simulink model "IEEE13bus_1subsystem"  (R2022b)
settings: Solver=ode4  StartTime=0.0  StopTime=inf  FixedStep=Ts  MaxStep=1e-4  RelTol=1e-4
InitFcn:
  | a=1; % Loading Factor
  | Ts=50e-6;
  | % phase to sequence conversion of RXB matrices
  | c=1*exp(sqrt(-1)*(120*pi/180));
  | T=[1 1 1;1 c*c c;1 c c*c];
  | Tinv=1/3*[1 1 1;1 c c*c;1 c*c c];
  | 
  | % Simulation data for the IEEE 13 Node Test Feeder model
  | mi2km = 1.60934;%  miles to km conversion
  | ft2km = 0.0003048; % feet to km conversion
  | ms2F = 1*1e-6/(2*pi*60);% microsiemens to Farads conversion
  | 
  | 
  | %% Configuration 601
  | % Series Resitance and Reactance - ohm/mile
  | R_601 = [0.3465 0.1560 0.1580;0.1560 0.3375 0.1535;0.1580 0.1535 0.3414];
  | X_601 = [1.1079 0.5017 0.4236;0.5017 1.0478 0.3849;0.4236 0.3849 1.0348];
  | % charging susceptance - microsiemens/mile
  | B_601 = [6.2998 -1.9958 -1.2595;-1.9958 5.9597 -0.7417;-1.2595 -0.7417 5.6386];
  | 
  | R_601 = R_601/mi2km;
  | Rseq=Tinv*R_601*T;
  | R1_601=Rseq(2,2);R0_601=Rseq(1,1);
  | 
  | L_601 = (X_601/(2*pi*60))/mi2km;
  | Lseq=Tinv*L_601*T;
  | L1_601=Lseq(2,2);L0_601=Lseq(1,1);
  | 
  | C_601 =(B_601*ms2F)/mi2km;
  | Cseq=Tinv*C_601*T;
  | C1_601=Cseq(2,2);C0_601=Cseq(1,1);
  | 
  | %% Configuration 602 - series reactance - ohm/mile
  | R_602 = [0.7526 0.1580 0.1560;0.1580 0.7475 0.1535;0.1560 0.1535 0.7436];
  | X_602 = [1.1814 0.4236 0.5017;0.4236 1.1983 0.3849;0.5017 0.3849 1.2112];
  | % charging susceptance - microsiemens/mile
  | B_602 = [5.6990 -1.0817 -1.6905;-1.0817 5.1795 -0.6588;-1.6905 -0.6588 5.4246];
  | 
  | R_602 = R_602/mi2km;
  | Rseq=Tinv*R_602*T;
  | R1_602=Rseq(2,2);R0_602=Rseq(1,1);
  | 
  | L_602 = (X_602/(2*pi*60))/mi2km;
  | Lseq=Tinv*L_602*T;
  | L1_602=Lseq(2,2);L0_602=Lseq(1,1);
  | 
  | C_602 =(B_602*ms2F)/mi2km;
  | Cseq=Tinv*C_602*T;
  | C1_602=Cseq(2,2);C0_602=Cseq(1,1);
  | %% Configuration 603 - series reactance - ohm/mile
  | R_603 = [0 0 0;0 1.3294 0.2066;0 0.2066 1.3238];
  | X_603 = [0 0 0;0 1.3471 0.4591;0 0.4591 1.3569];
  | % charging susceptance - microsiemens/mile
  | B_603 = [0 0 0;0 4.7097 -0.8999;0 -0.8999 4.6658];
  | 
  | % convert for SPS
  | R_603 = R_603/mi2km;
  | Rseq=Tinv*R_603*T;
  | R1_603=Rseq(2,2);R0_603=Rseq(1,1);
  | 
  | ... (+71 lines)
undefined symbols (not defined in the file): find_system, I, Left, MOV_segment9, powergui, Right, type, V, X
libraries: spsSeriesRLCBranchLib x57, spsGroundLib x42, spsVoltageMeasurementLib x18, spsThreePhaseVIMeasurementLib x16, spsDCVoltageSourceLib x12, spsThreePhaseSeriesRLCLoadLib x7, ssn_lib x6, spsACCurrentSourceLib x6, spsOnDelayLib x6, spsThreePhasePISectionLineLib x5, spsSeriesRLCLoadLib x5, spsRMSLib x4
(part 2 of 4)

== system IEEE13bus_1subsystem/SM_13p/Regulator 1 ==
  Mux : Mux  Inputs=3
  Single Phase SVR_A : Subsystem  LoadFcn=find_system(gcs,'FollowLinks', 'on', 'LookUnderMasks', 'all');  mask(Single-Phase OLTC){pNom=5e6/3, fNom=60, vNom=4160/sqrt(3), ctRatio=700, ptRatio=20, DeltaU=0.00625, TapMinMax=[-16 16], InitialTap=10, TapSelectionTime=0.2, RegulatorOn=on, Regulator=[122/120  2/120  0.2], Comp=[3 9]}
      mask prompts: pNom "Nominal Power (VA)"; fNom "Nominal Frequency (Hz)"; vNom "Nominal Voltage (Vrms)"; ctRatio "Primary CT Rating (A)"; ptRatio "PT Ratio"; DeltaU "Voltage Step Per Tap (pu)"; TapMinMax "Minimum and Maximum Tap Positions"; InitialTap "Initial Tap Position"; TapSelectionTime "Tap Selection Time (s)"; RegulatorOn "Voltage Regulator"; Regulator "Voltage Regulator [ Vref(pu) DeadBand(pu)  Delay(s)]"; Comp "Compensator Settings [R (V) X(V)]"
      mask help:
      | Models a single-phase On Load Tap Changer (OLTC). The single-phase secondary of multi-tap winding is modeled with a Variable-Ratio Transformer block.
      |
      | The transformer voltage ratio U2/U1 (in pu) is given by:
      |                 U2/U1= 1+TapPosition*DeltaU
      | Tap position 0 corresponds to nominal voltage ratio.
      |
      | When Voltage regulator is 'on',  voltage regulator asks for a tap change if:
      |                  abs(Vm-Vref)>DeadBand/2  during a time  t > Delay.
      |
      | where 'Vm' is voltage measured at regulating point and Vref is reference voltage.
      | With line drop compensation, Vm=Vsec-Isec(R+jX)
      mask init:
      | RegulatorVref=Regulator(1);
      | RegulatorDeadBand=Regulator(2);
      | RegulatorDelay=Regulator(3);
      | Rc=Comp(1);
      | Xc=Comp(2);
      mask TypeOptions RegulatorOn: off | on
      mask Callback RegulatorOn:
      | tempMaskVis=get_param(gcb,'MaskVisibilities');
      | if strcmp(get_param(gcb,'RegulatorOn'),'on')
      | 	tempMaskVis{11}='on';
      | 	set_param(gcb,'MaskVisibilities',tempMaskVis);
      | else
      | 	tempMaskVis{11}='off';
      | 	set_param(gcb,'MaskVisibilities',tempMaskVis);
      | end
      | if strcmp(get_param(gcb,'RegulatorOn'),'on')
      | 	tempMaskVis{12}='on';
      | 	set_param(gcb,'MaskVisibilities',tempMaskVis);
      | else
      | 	tempMaskVis{12}='off';
      | 	set_param(gcb,'MaskVisibilities',tempMaskVis);
      | end
      mask DialogControl Container8 Prompt: Setup
      mask DialogControl Container13 Prompt: Regulator Parameters
      mask Display:
      | color('green');
      | r=50;x=40;y=80;
      | th = 0:pi/100:2*pi;
      | f = r * exp(j*th) + x+j*y;
      | plot(real(f), imag(f));
      | color('blue');
      | plot([-10 90],[30,130])
      | plot([75 90],[125,130])
      | plot([85 90],[115,130])
      | color('black')
      | port_label('Lconn',1,'S');port_label('Rconn',1,'L');
      | text(58,115,'Tap');
      | text(43,70,'Vsec');
      | text(48,95,'Isec');
  Single Phase SVR_A1 : Subsystem  LoadFcn=find_system(gcs,'FollowLinks', 'on', 'LookUnderMasks', 'all');  mask(Single-Phase OLTC){pNom=5e6/3, fNom=60, vNom=4160/sqrt(3), ctRatio=700, ptRatio=20, DeltaU=0.00625, TapMinMax=[-16 16], InitialTap=8, TapSelectionTime=0.2, RegulatorOn=on, Regulator=[122/120  2/120  0.2], Comp=[3 9]}
      mask prompts: pNom "Nominal Power (VA)"; fNom "Nominal Frequency (Hz)"; vNom "Nominal Voltage (Vrms)"; ctRatio "Primary CT Rating (A)"; ptRatio "PT Ratio"; DeltaU "Voltage Step Per Tap (pu)"; TapMinMax "Minimum and Maximum Tap Positions"; InitialTap "Initial Tap Position"; TapSelectionTime "Tap Selection Time (s)"; RegulatorOn "Voltage Regulator"; Regulator "Voltage Regulator [ Vref(pu) DeadBand(pu)  Delay(s)]"; Comp "Compensator Settings [R (V) X(V)]"
      mask help:
      | Models a single-phase On Load Tap Changer (OLTC). The single-phase secondary of multi-tap winding is modeled with a Variable-Ratio Transformer block.
      |
      | The transformer voltage ratio U2/U1 (in pu) is given by:
      |                 U2/U1= 1+TapPosition*DeltaU
      | Tap position 0 corresponds to nominal voltage ratio.
      |
      | When Voltage regulator is 'on',  voltage regulator asks for a tap change if:
      |                  abs(Vm-Vref)>DeadBand/2  during a time  t > Delay.
      |
      | where 'Vm' is voltage measured at regulating point and Vref is reference voltage.
      | With line drop compensation, Vm=Vsec-Isec(R+jX)
      mask init:
      | RegulatorVref=Regulator(1);
      | RegulatorDeadBand=Regulator(2);
      | RegulatorDelay=Regulator(3);
      | Rc=Comp(1);
      | Xc=Comp(2);
      mask TypeOptions RegulatorOn: off | on
      mask Callback RegulatorOn:
      | tempMaskVis=get_param(gcb,'MaskVisibilities');
      | if strcmp(get_param(gcb,'RegulatorOn'),'on')
      | 	tempMaskVis{11}='on';
      | 	set_param(gcb,'MaskVisibilities',tempMaskVis);
      | else
      | 	tempMaskVis{11}='off';
      | 	set_param(gcb,'MaskVisibilities',tempMaskVis);
      | end
      | if strcmp(get_param(gcb,'RegulatorOn'),'on')
      | 	tempMaskVis{12}='on';
      | 	set_param(gcb,'MaskVisibilities',tempMaskVis);
      | else
      | 	tempMaskVis{12}='off';
      | 	set_param(gcb,'MaskVisibilities',tempMaskVis);
      | end
      mask DialogControl Container8 Prompt: Setup
      mask DialogControl Container13 Prompt: Regulator Parameters
      mask Display:
      | color('green');
      | r=50;x=40;y=80;
      | th = 0:pi/100:2*pi;
      | f = r * exp(j*th) + x+j*y;
      | plot(real(f), imag(f));
      | color('blue');
      | plot([-10 90],[30,130])
      | plot([75 90],[125,130])
      | plot([85 90],[115,130])
      | color('black')
      | port_label('Lconn',1,'S');port_label('Rconn',1,'L');
      | text(58,115,'Tap');
      | text(43,70,'Vsec');
      | text(48,95,'Isec');
  Single Phase SVR_A2 : Subsystem  LoadFcn=find_system(gcs,'FollowLinks', 'on', 'LookUnderMasks', 'all');  mask(Single-Phase OLTC){pNom=5e6/3, fNom=60, vNom=4160/sqrt(3), ctRatio=700, ptRatio=20, DeltaU=0.00625, TapMinMax=[-16 16], InitialTap=11, TapSelectionTime=0.2, RegulatorOn=on, Regulator=[122/120  2/120  0.2], Comp=[3 9]}
      mask prompts: pNom "Nominal Power (VA)"; fNom "Nominal Frequency (Hz)"; vNom "Nominal Voltage (Vrms)"; ctRatio "Primary CT Rating (A)"; ptRatio "PT Ratio"; DeltaU "Voltage Step Per Tap (pu)"; TapMinMax "Minimum and Maximum Tap Positions"; InitialTap "Initial Tap Position"; TapSelectionTime "Tap Selection Time (s)"; RegulatorOn "Voltage Regulator"; Regulator "Voltage Regulator [ Vref(pu) DeadBand(pu)  Delay(s)]"; Comp "Compensator Settings [R (V) X(V)]"
      mask help:
      | Models a single-phase On Load Tap Changer (OLTC). The single-phase secondary of multi-tap winding is modeled with a Variable-Ratio Transformer block.
      |
      | The transformer voltage ratio U2/U1 (in pu) is given by:
      |                 U2/U1= 1+TapPosition*DeltaU
      | Tap position 0 corresponds to nominal voltage ratio.
      |
      | When Voltage regulator is 'on',  voltage regulator asks for a tap change if:
      |                  abs(Vm-Vref)>DeadBand/2  during a time  t > Delay.
      |
      | where 'Vm' is voltage measured at regulating point and Vref is reference voltage.
      | With line drop compensation, Vm=Vsec-Isec(R+jX)
      mask init:
      | RegulatorVref=Regulator(1);
      | RegulatorDeadBand=Regulator(2);
      | RegulatorDelay=Regulator(3);
      | Rc=Comp(1);
      | Xc=Comp(2);
      mask TypeOptions RegulatorOn: off | on
      mask Callback RegulatorOn:
      | tempMaskVis=get_param(gcb,'MaskVisibilities');
      | if strcmp(get_param(gcb,'RegulatorOn'),'on')
      | 	tempMaskVis{11}='on';
      | 	set_param(gcb,'MaskVisibilities',tempMaskVis);
      | else
      | 	tempMaskVis{11}='off';
      | 	set_param(gcb,'MaskVisibilities',tempMaskVis);
      | end
      | if strcmp(get_param(gcb,'RegulatorOn'),'on')
      | 	tempMaskVis{12}='on';
      | 	set_param(gcb,'MaskVisibilities',tempMaskVis);
      | else
      | 	tempMaskVis{12}='off';
      | 	set_param(gcb,'MaskVisibilities',tempMaskVis);
      | end
      mask DialogControl Container8 Prompt: Setup
      mask DialogControl Container13 Prompt: Regulator Parameters
      mask Display:
      | color('green');
      | r=50;x=40;y=80;
      | th = 0:pi/100:2*pi;
      | f = r * exp(j*th) + x+j*y;
      | plot(real(f), imag(f));
      | color('blue');
      | plot([-10 90],[30,130])
      | plot([75 90],[125,130])
      | plot([85 90],[115,130])
      | color('black')
      | port_label('Lconn',1,'S');port_label('Rconn',1,'L');
      | text(58,115,'Tap');
      | text(43,70,'Vsec');
      | text(48,95,'Isec');
  A : PMIOPort  Side=Left
  a : PMIOPort  Port=2  Side=Right
  B : PMIOPort  Port=3  Side=Left
  b : PMIOPort  Port=4  Side=Right
  C : PMIOPort  Port=5  Side=Left
  c : PMIOPort  Port=6  Side=Right
  Tap : Outport
  wires:
  Single Phase SVR_A/1(Tap) -> Mux/1
  Single Phase SVR_A1/1(Tap) -> Mux/2
  Single Phase SVR_A2/1(Tap) -> Mux/3
  Mux/1 -> Tap/1
  connections:
  Single Phase SVR_A/RConn1 -- a/RConn1
  Single Phase SVR_A/LConn1 -- A/RConn1
  Single Phase SVR_A1/LConn1 -- B/RConn1
  Single Phase SVR_A1/RConn1 -- b/RConn1
  Single Phase SVR_A2/LConn1 -- C/RConn1
  Single Phase SVR_A2/RConn1 -- c/RConn1

== system IEEE13bus_1subsystem/SM_13p/Regulator Taps  ==
  Band Width : Constant  Value=2
  Band Width1 : Constant  Value=2
  Gain : Gain  Gain=1/2
  Gain2 : Gain  Gain=1/2
  Scope3 : Scope  NumInputPorts=5
  Sum : Sum  Inputs=|++
  Sum1 : Sum  Inputs=|+-
  Tap : Scope
  Vref : Constant  Value=122
  Vref1 : Constant  Value=122
  wires:
  [Rg1] -> Tap/1
  Vref/1 -> Sum/1
  Band Width/1 -> Gain/1
  Gain/1 -> Sum/2
  Gain2/1 -> Sum1/2
  Band Width1/1 -> Gain2/1
  Vref1/1 -> Sum1/1
  Sum/1 -> Scope3/1  "Upper Limit"
  [Vr1a] -> Scope3/2  "Vra"
  [Vr1b] -> Scope3/3  "Vrb"
  [Vr1c] -> Scope3/4  "Vrc"
  Sum1/1 -> Scope3/5  "Lower Limit"

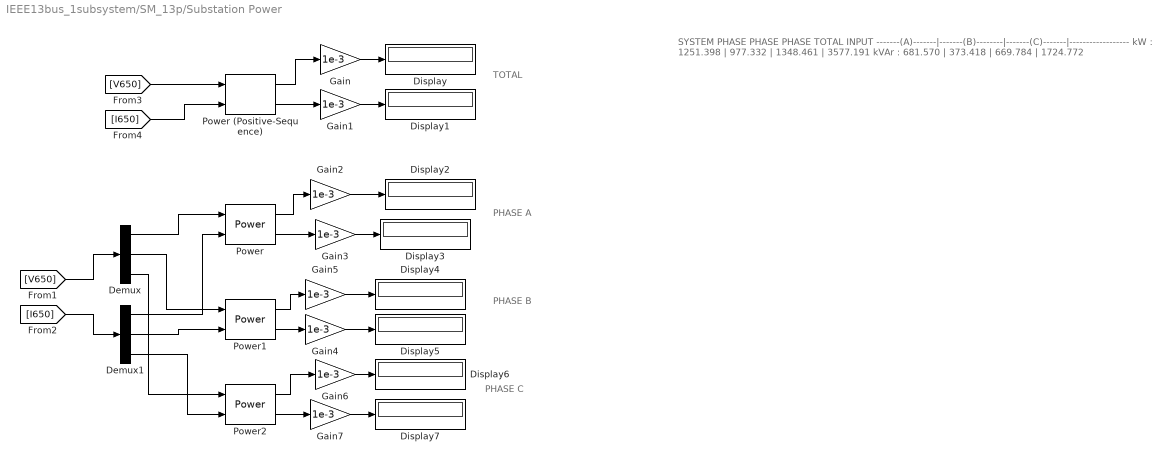
== system IEEE13bus_1subsystem/SM_13p/Substation Power ==
  note: SYSTEM PHASE PHASE PHASE TOTAL
      | INPUT -------(A)-------|-------(B)--------|-------(C)-------|------------------
      | kW : 1251.398 | 977.332 | 1348.461 | 3577.191
      | kVAr : 681.570 | 373.418 | 669.784 | 1724.772
  note: PHASE A
  note: PHASE C
  note: PHASE B
  note: TOTAL
  Demux : Demux  Outputs=3
  Demux1 : Demux  Outputs=3
  Display{,1..7} (8 alike) : Display
  Gain{,1..7} (8 alike) : Gain  Gain=1e-3
  Power : spsPowerLib/Power  Freq=60  Vinit=[1, 0]  Iinit=[1, 0]  Ts=0
  Power (Positive-Sequence) : spsPowerPositiveSequenceLib/Power (Positive-Sequence)  Freq=60  Vinit=[0, 0]  Iinit=[0, 0]  Ts=Ts
      settings: LibrarySourceBlock=|
      | sps_lib/Sensors and Measurements/Power
      | (Positive-Sequence)
  Power1 : spsPowerLib/Power  Freq=60  Vinit=[1, 0]  Iinit=[1, 0]  Ts=0
  Power2 : spsPowerLib/Power  Freq=60  Vinit=[1, 0]  Iinit=[1, 0]  Ts=0
  wires:
  [I650] -> Power (Positive-Sequence)/2
  [V650] -> Power (Positive-Sequence)/1
  Power (Positive-Sequence)/1 -> Gain/1
  Power (Positive-Sequence)/2 -> Gain1/1
  [V650] -> Demux/1
  [I650] -> Demux1/1
  Demux/1 -> Power/1
  Demux1/1 -> Power/2
  Demux/2 -> Power1/1
  Demux1/2 -> Power1/2
  Demux/3 -> Power2/1
  Demux1/3 -> Power2/2
  Power/1 -> Gain2/1
  Power/2 -> Gain3/1
  Power1/1 -> Gain5/1
  Power1/2 -> Gain4/1
  Power2/1 -> Gain6/1
  Power2/2 -> Gain7/1
  Gain/1 -> Display/1
  Gain1/1 -> Display1/1
  Gain2/1 -> Display2/1
  Gain3/1 -> Display3/1
  Gain4/1 -> Display5/1
  Gain5/1 -> Display4/1
  Gain6/1 -> Display6/1
  Gain7/1 -> Display7/1

== system IEEE13bus_1subsystem/powergui/EquivalentModel1 ==
  Sources : Subsystem
  State-Space : S-Function  FunctionName=ssn_sfun_v1  Parameters=1,0  SFunctionDeploymentMode=off  EnableBusSupport=off  SFcnStateName=MOV_segment9,MOV_segment9,MOV_segment9,MOV_segment9,MOV_segment9,MOV_segment9,MOV_segment9,MOV_segment9,MOV_segment9,MOV_segment9
      settings: SFcnIsStateOwnerBlock=on
  Yout : Subsystem
  wires:
  State-Space/1 -> Yout/1(v,i)
  Sources/1(u) -> State-Space/1

== system IEEE13bus_1subsystem/powergui/EquivalentModel2 ==
  Sources : Subsystem
  State-Space : S-Function  FunctionName=ssn_sfun_v1  Parameters=2,0  SFunctionDeploymentMode=off  EnableBusSupport=off  SFcnStateName=MOV_segment9,MOV_segment9,MOV_segment9,MOV_segment9,MOV_segment9,MOV_segment9,MOV_segment9,MOV_segment9,MOV_segment9,MOV_segment9
      settings: SFcnIsStateOwnerBlock=on
  Yout : Subsystem
  wires:
  State-Space/1 -> Yout/1(v,i)
  Sources/1(u) -> State-Space/1

== system IEEE13bus_1subsystem/powergui/EquivalentModel3 ==
  Sources : Subsystem
  State-Space : S-Function  FunctionName=ssn_sfun_v1  Parameters=3,0  SFunctionDeploymentMode=off  EnableBusSupport=off  SFcnStateName=MOV_segment9,MOV_segment9,MOV_segment9,MOV_segment9,MOV_segment9,MOV_segment9,MOV_segment9,MOV_segment9,MOV_segment9,MOV_segment9
      settings: SFcnIsStateOwnerBlock=on
  Yout : Subsystem
  wires:
  State-Space/1 -> Yout/1(v,i)
  Sources/1(u) -> State-Space/1

== system IEEE13bus_1subsystem/powergui/EquivalentModel4 ==
  Gates : Subsystem
  Sources : Subsystem
  State-Space : Subsystem
  Status : Subsystem
  Yout : Subsystem
  wires:
  Gates/1(gates) -> State-Space/2(In2)
  Sources/1(u) -> State-Space/1(In1)
  State-Space/2(Out2) -> Status/1(status)
  State-Space/1(Out1) -> Yout/1(v,i)

== system IEEE13bus_1subsystem/SM_13p/Regulator 1/Single Phase SVR_A ==
  Line Drop Compensator : Subsystem
  Transformer with Taps : Subsystem
  Voltage Regulator Control : Subsystem
  S : PMIOPort  Tag=PMCPort  Side=Left
  L : PMIOPort  Tag=PMCPort  Port=2  Side=Right
  Tap : Outport  VectorParamsAs1DForOutWhenUnconnected=off
  tag scope: Vr1a=global
  wires:
  Transformer with Taps/2(Vsec) -> Line Drop Compensator/2(Vsec)
  Transformer with Taps/1(Isec) -> Line Drop Compensator/1(Isec)
  Voltage Regulator Control/1(N) -> Transformer with Taps/1(N)
  Voltage Regulator Control/2(Tap) -> Tap/1
  Line Drop Compensator/1(Vm) -> [Vr1a], Voltage Regulator Control/1(Vm)
  connections:
  Transformer with Taps/LConn1 -- S/RConn1
  Transformer with Taps/RConn1 -- L/RConn1

== system IEEE13bus_1subsystem/SM_13p/Regulator 1/Single Phase SVR_A1 ==
  Line Drop Compensator : Subsystem
  Transformer with Taps : Subsystem
  Voltage Regulator Control : Subsystem
  S : PMIOPort  Tag=PMCPort  Side=Left
  L : PMIOPort  Tag=PMCPort  Port=2  Side=Right
  Tap : Outport  VectorParamsAs1DForOutWhenUnconnected=off
  tag scope: Vr1b=global
  wires:
  Line Drop Compensator/1(Vm) -> Voltage Regulator Control/1(Vm), [Vr1b]
  Voltage Regulator Control/2(Tap) -> Tap/1
  Voltage Regulator Control/1(N) -> Transformer with Taps/1(N)
  Transformer with Taps/1(Isec) -> Line Drop Compensator/1(Isec)
  Transformer with Taps/2(Vsec) -> Line Drop Compensator/2(Vsec)
  connections:
  Transformer with Taps/RConn1 -- L/RConn1
  Transformer with Taps/LConn1 -- S/RConn1

== system IEEE13bus_1subsystem/SM_13p/Regulator 1/Single Phase SVR_A2 ==
  Line Drop Compensator : Subsystem
  Transformer with Taps : Subsystem
  Voltage Regulator Control : Subsystem
  S : PMIOPort  Tag=PMCPort  Side=Left
  L : PMIOPort  Tag=PMCPort  Port=2  Side=Right
  Tap : Outport  VectorParamsAs1DForOutWhenUnconnected=off
  tag scope: Vr1c=global
  wires:
  Transformer with Taps/2(Vsec) -> Line Drop Compensator/2(Vsec)
  Transformer with Taps/1(Isec) -> Line Drop Compensator/1(Isec)
  Voltage Regulator Control/1(N) -> Transformer with Taps/1(N)
  Voltage Regulator Control/2(Tap) -> Tap/1
  Line Drop Compensator/1(Vm) -> [Vr1c], Voltage Regulator Control/1(Vm)
  connections:
  Transformer with Taps/LConn1 -- S/RConn1
  Transformer with Taps/RConn1 -- L/RConn1

== system IEEE13bus_1subsystem/powergui/EquivalentModel1/Sources ==
  Mux : Mux  Inputs=[1 1]
  u : Outport  VectorParamsAs1DForOutWhenUnconnected=off
  wires:
  Mux/1 -> u/1
  [T91_7966_12561094007631] -> Mux/1
  [T91_7953_12480495761568] -> Mux/2

== system IEEE13bus_1subsystem/powergui/EquivalentModel1/Yout ==
  v,i : Inport
  Demux : Demux  Outputs=1
  tag scope: T94_8498_15482413429189=global
  wires:
  v,i/1 -> Demux/1
  Demux/1 -> [T94_8498_15482413429189]

== system IEEE13bus_1subsystem/powergui/EquivalentModel2/Sources ==
  Mux : Mux  Inputs=[1 1]
  u : Outport  VectorParamsAs1DForOutWhenUnconnected=off
  wires:
  Mux/1 -> u/1
  [T92_8015_12801519000204] -> Mux/1
  [T92_8002_12718661753869] -> Mux/2

== system IEEE13bus_1subsystem/powergui/EquivalentModel2/Yout ==
  v,i : Inport
  Demux : Demux  Outputs=1
  tag scope: T95_8547_15793615812972=global
  wires:
  v,i/1 -> Demux/1
  Demux/1 -> [T95_8547_15793615812972]

== system IEEE13bus_1subsystem/powergui/EquivalentModel3/Sources ==
  Mux : Mux  Inputs=[1 1]
  u : Outport  VectorParamsAs1DForOutWhenUnconnected=off
  wires:
  Mux/1 -> u/1
  [T92_8016_12799101659306] -> Mux/1
  [T92_8003_12716269942909] -> Mux/2

== system IEEE13bus_1subsystem/powergui/EquivalentModel3/Yout ==
  v,i : Inport
  Demux : Demux  Outputs=1
  tag scope: T95_8548_15790470056233=global
  wires:
  v,i/1 -> Demux/1
  Demux/1 -> [T95_8548_15790470056233]

== system IEEE13bus_1subsystem/powergui/EquivalentModel4/Gates ==
  Mux : Mux  Inputs=[1 1 1 1 1 1]
  gates : Outport  VectorParamsAs1DForOutWhenUnconnected=off
  wires:
  Mux/1 -> gates/1
  [T62_5500_5957741646095] -> Mux/1
  [T62_5501_5960629368675] -> Mux/2
  [T62_5502_5963692782869] -> Mux/3
  [T58_5116_5284246709138] -> Mux/4
  [T58_5117_5286921221031] -> Mux/5
  [T58_5118_5289758007408] -> Mux/6

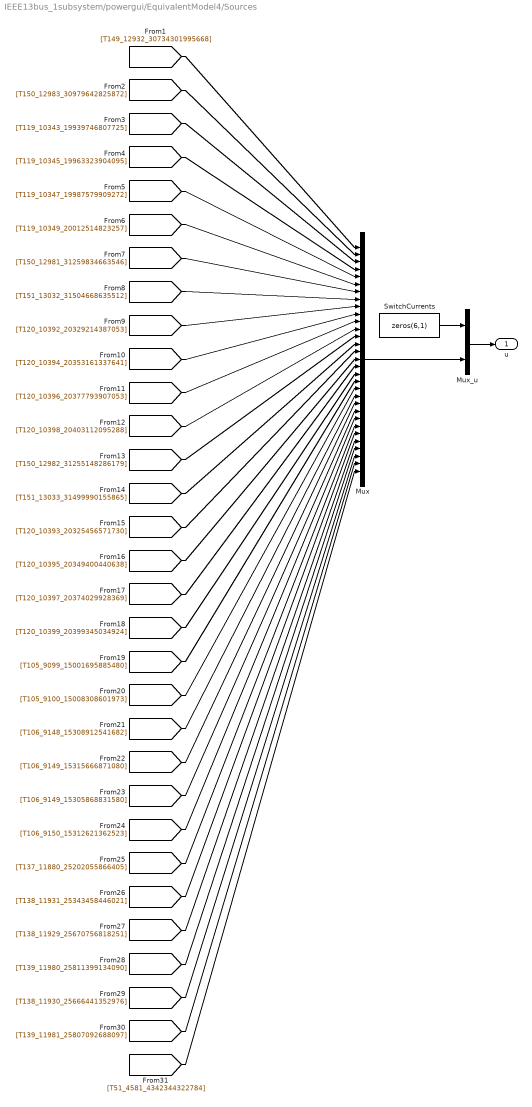
== system IEEE13bus_1subsystem/powergui/EquivalentModel4/Sources ==
  Mux : Mux  Inputs=[1 1 1 1 1 1 1 1 1 1 1 1 1 1 1 1 1 1 1 1 1 1 1 1 1 1 1 1 1 1 3]
  Mux_u : Mux  Inputs=[6 33]
  SwitchCurrents : Constant  Value=zeros(6,1)
  u : Outport  VectorParamsAs1DForOutWhenUnconnected=off
  wires:
  Mux_u/1 -> u/1
  SwitchCurrents/1 -> Mux_u/1
  Mux/1 -> Mux_u/2
  [T149_12932_30734301995668] -> Mux/1
  [T150_12983_30979642825872] -> Mux/2
  [T119_10343_19939746807725] -> Mux/3
  [T119_10345_19963323904095] -> Mux/4
  [T119_10347_19987579909272] -> Mux/5
  [T119_10349_20012514823257] -> Mux/6
  [T150_12981_31259834663546] -> Mux/7
  [T151_13032_31504668635512] -> Mux/8
  [T120_10392_20329214387053] -> Mux/9
  [T120_10394_20353161337641] -> Mux/10
  [T120_10396_20377793907053] -> Mux/11
  [T120_10398_20403112095288] -> Mux/12
  [T150_12982_31255148286179] -> Mux/13
  [T151_13033_31499990155865] -> Mux/14
  [T120_10393_20325456571730] -> Mux/15
  [T120_10395_20349400440638] -> Mux/16
  [T120_10397_20374029928369] -> Mux/17
  [T120_10399_20399345034924] -> Mux/18
  [T105_9099_15001695885480] -> Mux/19
  [T105_9100_15008308601973] -> Mux/20
  [T106_9148_15308912541682] -> Mux/21
  [T106_9149_15315666871080] -> Mux/22
  [T106_9149_15305868831580] -> Mux/23
  [T106_9150_15312621362523] -> Mux/24
  [T137_11880_25202055866405] -> Mux/25
  [T138_11931_25343458446021] -> Mux/26
  [T138_11929_25670756818251] -> Mux/27
  [T139_11980_25811399134090] -> Mux/28
  [T138_11930_25666441352976] -> Mux/29
  [T139_11981_25807092688097] -> Mux/30
  [T51_4581_4342344322784] -> Mux/31

== system IEEE13bus_1subsystem/powergui/EquivalentModel4/State-Space ==
  In1 : Inport
  In2 : Inport  Port=2
  ssn_sfun_sw1 : S-Function  FunctionName=ssn_sfun_v1  Parameters=4,0  SFunctionDeploymentMode=off  EnableBusSupport=off  SFcnStateName=MOV_segment49,xn_g1,xn_g2,xn_g3,xn_g4,MOV_segment49,MOV_segment49,MOV_segment49,MOV_segment49,MOV_segment49,MOV_segment49,MOV_segment49,MOV_segment49,MOV_segment49,MOV_segment49,MOV_segment49,MOV_segment49,MOV_segment49,MOV_segment49,MOV_segment49,MOV_segment49,MOV_segment49,MOV_segment49,MOV_segment49,MOV_segment49,MOV_segment49,MOV_segment49,MOV_segment49,MOV_segment49,MOV_segment49,MOV_segment49,MOV_segment49,MOV_segment49,MOV_segment49,MOV_segment49,MOV_segment49,MOV_segment49,MOV_segment49,MOV_segment49,MOV_segment49,MOV_segment49,MOV_segment49,MOV_segment49,MOV_segment49,MOV_segment49,MOV_segment49,MOV_segment49,MOV_segment49,MOV_segment49,MOV_segment49
      settings: SFcnIsStateOwnerBlock=on
  Out1 : Outport  VectorParamsAs1DForOutWhenUnconnected=off
  Out2 : Outport  Port=2  VectorParamsAs1DForOutWhenUnconnected=off
  tag scope: ssn_ext_sys_from_V_39cxbf7cx045ce1b35499=global, ssn_ext_sys_from_V_3eaxbe2ex28c4bec03d51=global, ssn_ext_sys_from_V_53dx83dbx55ea16c77358=global
  wires:
  ssn_sfun_sw1/2 -> Out2/1
  In2/1 -> ssn_sfun_sw1/2
  ssn_sfun_sw1/1 -> Out1/1
  In1/1 -> ssn_sfun_sw1/1
  [ssn_ext_sys_goto_Hist_53dx83dbx55ea16c77358] -> ssn_sfun_sw1/3
  [ssn_ext_sys_goto_Y_53dx83dbx55ea16c77358] -> ssn_sfun_sw1/4
  ssn_sfun_sw1/3 -> [ssn_ext_sys_from_V_53dx83dbx55ea16c77358]
  [ssn_ext_sys_goto_Hist_39cxbf7cx045ce1b35499] -> ssn_sfun_sw1/5
  [ssn_ext_sys_goto_Y_39cxbf7cx045ce1b35499] -> ssn_sfun_sw1/6
  ssn_sfun_sw1/4 -> [ssn_ext_sys_from_V_39cxbf7cx045ce1b35499]
  [ssn_ext_sys_goto_Hist_3eaxbe2ex28c4bec03d51] -> ssn_sfun_sw1/7
  [ssn_ext_sys_goto_Y_3eaxbe2ex28c4bec03d51] -> ssn_sfun_sw1/8
  ssn_sfun_sw1/5 -> [ssn_ext_sys_from_V_3eaxbe2ex28c4bec03d51]

== system IEEE13bus_1subsystem/powergui/EquivalentModel4/Status ==
  status : Inport
  Demux : Demux  Outputs=[1 1 1 1 1 1]
  tag scope: T60_5351_6088299148023=global, T60_5352_6090445037412=global, T60_5353_6092747792136=global, T64_5735_6809575442857=global, T64_5736_6811932002054=global, T64_5737_6814458762500=global
  wires:
  status/1 -> Demux/1
  Demux/1 -> [T64_5735_6809575442857]
  Demux/2 -> [T64_5736_6811932002054]
  Demux/3 -> [T64_5737_6814458762500]
  Demux/4 -> [T60_5351_6088299148023]
  Demux/5 -> [T60_5352_6090445037412]
  Demux/6 -> [T60_5353_6092747792136]

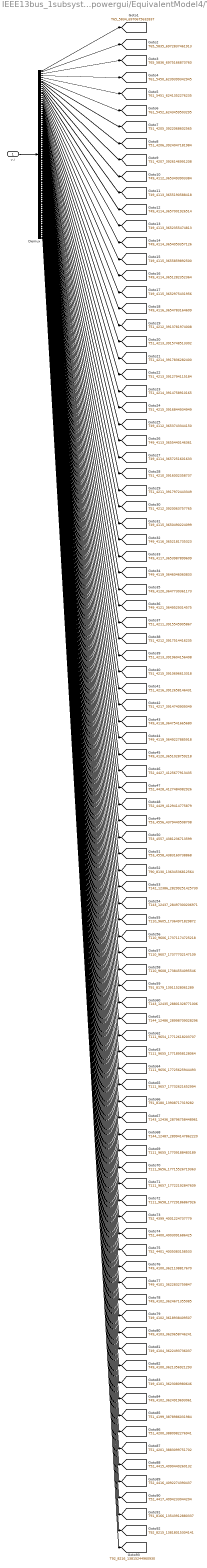
== system IEEE13bus_1subsystem/powergui/EquivalentModel4/Yout ==
  v,i : Inport
  Demux : Demux  Outputs=[1 1 1 1 1 1 1 1 1 1 1 1 1 1 1 1 1 1 1 1 1 1 1 1 1 1 1 1 1 1 1 1 1 1 1 1 1 1 1 1 1 1 1 1 1 1 1 1 1 1 1 1 1 1 1 1 1 1 1 1 1 1 1 1 1 1 1 1 1 1 1 1 1 1 1 1 1 1 1 1 1 1 1 1 1 1 1 1 1 1 1 1 1]
  tag scope: T110_9605_17364971829872=global, T110_9606_17371174725218=global, T110_9607_17377702147109=global, T110_9608_17384554095546=global, T111_9654_17712618203707=global, T111_9655_17709188483189=global, T111_9655_17718958128064=global, T111_9656_17715526719363=global, T111_9656_17725625944493=global, T111_9657_17722192847609=global, T111_9657_17732621652994=global, T111_9658_17729186867926=global, T142_12386_28299251425730=global, T143_12435_28801328771006=global, T143_12436_28796758448961=global, T143_12437_28497300206971=global, T144_12486_28998709028296=global, T144_12487_28994147862220=global, T49_4100_3621108817670=global, T49_4100_3621356921293=global, T49_4101_3622832759847=global, T49_4101_3623080980646=global, T49_4102_3618938409507=global, T49_4102_3624671355085=global, T49_4102_3624919693061=global, T49_4103_3620658746241=global, T49_4104_3622493736037=global, T49_4112_3653493903384=global, T49_4112_3653743344150=global, T49_4113_3652355474813=global, T49_4113_3655190588418=global, T49_4113_3655440146361=global, T49_4114_3651282352364=global, T49_4114_3654050357126=global, T49_4114_3657001926514=global, T49_4114_3657251601633=global, T49_4115_3650490224099=global, T49_4115_3652975431956=global, T49_4115_3655859892500=global, T49_4116_3652181735323=global, T49_4116_3654783164609=global, T49_4117_3653987899609=global, T49_4118_3647541665680=global, T49_4119_3646046060833=global, T49_4119_3649227885918=global, T49_4120_3647730361173=global, T49_4120_3651028759218=global, T49_4121_3649529314575=global, T51_4199_3878986031984=global, T51_4200_3880982276941=global, T51_4201_3883099751702=global, T51_4205_3922068602565=global, T51_4206_3924047181984=global, T51_4207_3926146991208=global, T51_4210_3916002358737=global, T51_4211_3915545905867=global, T51_4211_3917972443349=global, T51_4212_3913781974008=global, T51_4212_3917514416235=global, T51_4212_3920063757765=global, T51_4213_3912794115184=global, T51_4213_3915748513302=global, T51_4213_3919604156408=global, T51_4214_3914758910165=global, T51_4214_3917836282400=global, T51_4215_3910696613318=global, T51_4215_3916844934949=global, T51_4216_3912658146431=global, T51_4217_3914740909349=global, T52_4399_4001224737779=global, T52_4400_4003091686425=global, T52_4401_4005083158533=global, T52_4415_4090440260132=global, T52_4416_4092274390437=global, T52_4417_4094233044204=global, T52_4427_4125677913435=global, T52_4428_4127484082926=global, T52_4429_4129414775879=global, T53_4556_4379440508708=global, T53_4557_4381236713599=global, T53_4558_4383160738868=global, T61_5450_6239399342945=global, T61_5451_6241352276235=global, T61_5452_6243459503295=global, T65_5834_6970675632837=global, T65_5835_6972837461913=global, T65_5836_6975166873760=global, T90_8130_13634536812564=global, T91_8166_13543912880337=global, T91_8179_13911528061289=global, T91_8180_13908717319282=global, T92_8215_13818015304141=global, T92_8216_13815244960930=global
  wires:
  v,i/1 -> Demux/1
  Demux/1 -> [T65_5834_6970675632837]
  Demux/2 -> [T65_5835_6972837461913]
  Demux/3 -> [T65_5836_6975166873760]
  Demux/4 -> [T61_5450_6239399342945]
  Demux/5 -> [T61_5451_6241352276235]
  Demux/6 -> [T61_5452_6243459503295]
  Demux/7 -> [T51_4205_3922068602565]
  Demux/8 -> [T51_4206_3924047181984]
  Demux/9 -> [T51_4207_3926146991208]
  Demux/10 -> [T49_4112_3653493903384]
  Demux/11 -> [T49_4113_3655190588418]
  Demux/12 -> [T49_4114_3657001926514]
  Demux/13 -> [T49_4113_3652355474813]
  Demux/14 -> [T49_4114_3654050357126]
  Demux/15 -> [T49_4115_3655859892500]
  Demux/16 -> [T49_4114_3651282352364]
  Demux/17 -> [T49_4115_3652975431956]
  Demux/18 -> [T49_4116_3654783164609]
  Demux/19 -> [T51_4212_3913781974008]
  Demux/20 -> [T51_4213_3915748513302]
  Demux/21 -> [T51_4214_3917836282400]
  Demux/22 -> [T51_4213_3912794115184]
  Demux/23 -> [T51_4214_3914758910165]
  Demux/24 -> [T51_4215_3916844934949]
  Demux/25 -> [T49_4112_3653743344150]
  Demux/26 -> [T49_4113_3655440146361]
  Demux/27 -> [T49_4114_3657251601633]
  Demux/28 -> [T51_4210_3916002358737]
  Demux/29 -> [T51_4211_3917972443349]
  Demux/30 -> [T51_4212_3920063757765]
  Demux/31 -> [T49_4115_3650490224099]
  Demux/32 -> [T49_4116_3652181735323]
  Demux/33 -> [T49_4117_3653987899609]
  Demux/34 -> [T49_4119_3646046060833]
  Demux/35 -> [T49_4120_3647730361173]
  Demux/36 -> [T49_4121_3649529314575]
  Demux/37 -> [T51_4211_3915545905867]
  Demux/38 -> [T51_4212_3917514416235]
  Demux/39 -> [T51_4213_3919604156408]
  Demux/40 -> [T51_4215_3910696613318]
  Demux/41 -> [T51_4216_3912658146431]
  Demux/42 -> [T51_4217_3914740909349]
  Demux/43 -> [T49_4118_3647541665680]
  Demux/44 -> [T49_4119_3649227885918]
  Demux/45 -> [T49_4120_3651028759218]
  Demux/46 -> [T52_4427_4125677913435]
  Demux/47 -> [T52_4428_4127484082926]
  Demux/48 -> [T52_4429_4129414775879]
  Demux/49 -> [T53_4556_4379440508708]
  Demux/50 -> [T53_4557_4381236713599]
  Demux/51 -> [T53_4558_4383160738868]
  Demux/52 -> [T90_8130_13634536812564]
  Demux/53 -> [T142_12386_28299251425730]
  Demux/54 -> [T143_12437_28497300206971]
  Demux/55 -> [T110_9605_17364971829872]
  Demux/56 -> [T110_9606_17371174725218]
  Demux/57 -> [T110_9607_17377702147109]
  Demux/58 -> [T110_9608_17384554095546]
  Demux/59 -> [T91_8179_13911528061289]
  Demux/60 -> [T143_12435_28801328771006]
  Demux/61 -> [T144_12486_28998709028296]
  Demux/62 -> [T111_9654_17712618203707]
  Demux/63 -> [T111_9655_17718958128064]
  Demux/64 -> [T111_9656_17725625944493]
  Demux/65 -> [T111_9657_17732621652994]
  Demux/66 -> [T91_8180_13908717319282]
  Demux/67 -> [T143_12436_28796758448961]
  Demux/68 -> [T144_12487_28994147862220]
  Demux/69 -> [T111_9655_17709188483189]
  Demux/70 -> [T111_9656_17715526719363]
  Demux/71 -> [T111_9657_17722192847609]
  Demux/72 -> [T111_9658_17729186867926]
  Demux/73 -> [T52_4399_4001224737779]
  Demux/74 -> [T52_4400_4003091686425]
  Demux/75 -> [T52_4401_4005083158533]
  Demux/76 -> [T49_4100_3621108817670]
  Demux/77 -> [T49_4101_3622832759847]
  Demux/78 -> [T49_4102_3624671355085]
  Demux/79 -> [T49_4102_3618938409507]
  Demux/80 -> [T49_4103_3620658746241]
  Demux/81 -> [T49_4104_3622493736037]
  Demux/82 -> [T49_4100_3621356921293]
  Demux/83 -> [T49_4101_3623080980646]
  Demux/84 -> [T49_4102_3624919693061]
  Demux/85 -> [T51_4199_3878986031984]
  Demux/86 -> [T51_4200_3880982276941]
  Demux/87 -> [T51_4201_3883099751702]
  Demux/88 -> [T52_4415_4090440260132]
  Demux/89 -> [T52_4416_4092274390437]
  Demux/90 -> [T52_4417_4094233044204]
  Demux/91 -> [T91_8166_13543912880337]
  Demux/92 -> [T92_8215_13818015304141]
  Demux/93 -> [T92_8216_13815244960930]

== system IEEE13bus_1subsystem/SM_13p/Regulator 1/Single Phase SVR_A/Line Drop Compensator ==
  note: Vm=Vsec-Isec(Rc+jXc)
  Isec : Inport
  Vsec : Inport  Port=2
  "        " : spsLinearTransformerLib/Linear Transformer  UNITS=SI  NominalPower=[pNom fNom]  winding1=[vNom/ptRatio 1e-7 1e-8]  winding2=[vNom/ptRatio 1e-7 1e-8]  ThreeWindings=off  winding3=[3.15e+005 0.7938 0.084225]  RmLm=[1e5 1e5]  Measurements=None  DataType=on
  "CTS  " : spsControlledCurrentSourceLib/Controlled Current Source  Initialize=on  Source_Type=AC  Amplitude=0  Phase=0  Frequency=0  Measurements=None
  "PTS  " : spsControlledVoltageSourceLib/Controlled Voltage Source  Initialize=on  Source_Type=AC  Amplitude=0  Phase=0  Frequency=0  Measurements=None
  RMS : spsRMSLib/RMS  TrueRMS=on  Freq=60  RMSInit=120  Ts=0
  Raux : spsSeriesRLCBranchLib/Series RLC Branch  LConnTagsString=__new0  RConnTagsString=__new0  BranchType=R  Resistance=1e3  Inductance=1.6 / (120*pi)  SetiL0=off  InitialCurrent=0  Capacitance=1e-6  Setx0=off  InitialVoltage=0  Measurements=None
  Rc+jXc : spsSeriesRLCBranchLib/Series RLC Branch  LConnTagsString=__new0  RConnTagsString=__new0  BranchType=RL  Resistance=Rc  Inductance=Xc / (2*pi*fNom)  SetiL0=off  InitialCurrent=0  Capacitance=1e-6  Setx0=off  InitialVoltage=0  Measurements=None
  VRelay : spsVoltageMeasurementLib/Voltage Measurement  PhasorSimulation=off  OutputType=Complex  PSBequivalent=0
  Vm : Outport
  wires:
  Vsec/1 -> "PTS  "/1
  Isec/1 -> "CTS  "/1
  VRelay/1 -> RMS/1
  RMS/1 -> Vm/1
  connections:
  VRelay/LConn2 -- "PTS  "/LConn1
  "        "/LConn2 -- "CTS  "/LConn1 -- Raux/RConn1 -- Rc+jXc/RConn1
  "CTS  "/RConn1 -- "        "/LConn1 -- Rc+jXc/LConn1 -- Raux/LConn1
  "        "/RConn2 -- VRelay/LConn1
  "PTS  "/RConn1 -- "        "/RConn1

== system IEEE13bus_1subsystem/SM_13p/Regulator 1/Single Phase SVR_A/Transformer with Taps ==
  note: Vsec on Pt Ratio base
  note: Isec on CT Ratio base
  N : Inport
  "   " : Terminator
  "    " : Gain  Gain=1/ptRatio
  " 1" : Gain  Gain=-1/ctRatio
  Back-Euler : Constant
  CT1 : spsCurrentMeasurementLib/Current Measurement  PhasorSimulation=off  OutputType=Complex  PSBequivalent=0
  Fcn : Fcn  Expr=1+0.1*u(1)/16
  Ground1 : spsGroundLib/Ground  LConnTagsString=a
  Memory : Memory
  Memory1 : Memory
  Mux1 : Mux  Inputs=2
  PT : spsVoltageMeasurementLib/Voltage Measurement  PhasorSimulation=off  OutputType=Complex  PSBequivalent=0
  SSN Interface Block (1ph) : ssn_lib/SSN Interface Block (1ph)  nb_phase=1  nb_port=2  p1_type=I-type(Left)  p2_type=X-type(Right)  p3_type=V-type(Left)  p4_type=V-type(Left)  p5_type=V-type(Left)  p6_type=V-type(Left)  p7_type=V-type(Left)  p8_type=V-type(Left)  p9_type=V-type(Left)  p10_type=V-type(Left)  p11_type=V-type(Left)  p12_type=V-type(Left)  p13_type=V-type(Left)  p14_type=V-type(Left)  p15_type=V-type(Left)  p16_type=V-type(Left)  I_port_shunt_resistance=1e9
  SSN Interface Block (1ph)2 : ssn_lib/SSN Interface Block (1ph)  nb_phase=1  nb_port=2  p1_type=X-type(Left)  p2_type=I-type(Right)  p3_type=X-type(Left)  p4_type=V-type (Right)  p5_type=V-type(Left)  p6_type=V-type(Left)  p7_type=V-type(Left)  p8_type=V-type(Left)  p9_type=V-type(Left)  p10_type=V-type(Left)  p11_type=V-type(Left)  p12_type=V-type(Left)  p13_type=V-type(Left)  p14_type=V-type(Left)  p15_type=V-type(Left)  p16_type=V-type(Left)  I_port_shunt_resistance=1e9
  SSN OLTC xfo v2 : Subsystem  AncestorBlock=artemis/SSN/SSN OLTC/SSN OLTC xfo v2  mask(Norton-Type External Nodal Subsystem){nnode=2, taggg=53dx83dbx55ea16c77358, conntype=2 ports, RLpri=[1e-3 1e-4], Rcore=10000, ensat=off, Lcore=100, Lsat=1, phisat=100, Ts=Ts}
      mask prompts: nnode "Number of Electric nodes"; taggg "Unique Tag Identifier (automatic)"; conntype "Connection type"; RLpri "Primary winding resistance and inductance ([Ohms H])"; Rcore "Core Resistance (Ohms)"; ensat "Enable Saturation"; Lcore "Unsaturated magnetisation inductance (H)"; Lsat "Saturated magnetisation inductance (H)"; phisat "Flux saturation threshold (Weber)"; Ts "Sample Time (s)"
      mask help:
      | Continuously-variable On-Load Tapped Transformer (OLTC) (SSN Custom model)
      |
      | This block implements a 2 winding OLTC saturable transformer in SSN.
      | The model has a variable secondary inductance and resistance as well as turn-ratio.
      | The secondary winding is on the side marked with 'TAP'
      |
      | Mask parameters:
      |    Unique Tag Identifier: unique tag required by SSN to recknonize SSN external models
      |    Primary winding resistance and inductance ([Ohms H])
      |    Core Resistance (Ohms)
      |    Unsaturated magnetisation inductance (H): unsaturated core magnetization inductance
      |    Saturated magnetisation inductance (H): local inductance of the core in the saturated region
      |    Flux saturation threshold (Weber): flux saturation point
      |
      | Signal parameters:
      |
      | Signal inputs:
      |    1st sig: secondary winding resistance (Ohms)
      |    2nd sig: secondary winding inductance (H)
      |    3rd sig: transformer turn ratio k (V_secondary_tapped=k*V_primary)
      |    4th sig:  when set to 1, uses the Backward Euler method for solver. This can be used dynamically during simulation for example to damp numerical oscillations after switching events or after tap changes.
      |
      | Signals ouputs:
      |    1st signal: primary input current (A)
      |    2nd signal: secondary winding current (A)
      |    3rd signal: transformer flux (Wb)
      |
      | Saturation characteristic:
      |          flux
      |             ^              2
      |             |      1       *   <--- slope between point1 and point2 is Lsaturated
      |  phisat  |-----*  <---  this is the knee of flux=f(imag)
      |             |
      |             |
      |             |  <-----slope between origin and point1 is Lunsaturated
      |             *-------------------> imag
      mask init:
      | bloc=gcb;
      | taggg=get_param(bloc,'taggg');
      | conntyp=get_param(bloc,'conntype');
      | set_param([bloc '/FromV'],'GotoTag',['ssn_ext_sys_from_V_' taggg]);
      | set_param([bloc '/GotoHist'],'GotoTag',['ssn_ext_sys_goto_Hist_' taggg]);
      | set_param([bloc '/GotoY'],'GotoTag',['ssn_ext_sys_goto_Y_' taggg]);
      | 
      | R1=RLpri(1);
      | L1=RLpri(2);
      | 
      | if isequal(get_param(bloc,'ensat'),'off')
      |     phisat=1e20;
      | end
      | 
      | if isequal(conntyp,'4 ports')
      |     vin_sel=[1 2 3 4];
      |     Vinzeros=0;
      |     hist_sel=[1 2 3 4];
      |     a1=0;a2=0;a3=100;a4=100; b1=[7,34,40,33,31,33,40,33,31,33,40,33,31,33,40,34,7];b2=[30,30,34,42,40,37,45,52,50,47,54,62,59,57,65,70,70];b3=[93,67,60,67,70,67,60,67,70,67,60,67,70,67,60,67,93];b4=[30,30,34,42,40,37,45,52,50,47,54,62,60,57,65,70,70];
      |     c1=[20,20]*0;c2=[20,30]*0;c3=[27,14]*0;c4=[20,20]*0;c5=[24,17]*0;c6=[16,16]*0;c7=[22,19]*0;c8=[13,13]*0;c9=[80,80]*0;c10=[20,30]*0;c11=[88,74]*0;c12=[20,20]*0;c13=[85,77]*0;c14=[16,16]*0;c15=[81,79]*0;c16=[13,13]*0;
      |     %d1=[85,80];d2=[60,60];d3=[83,83];d4=[50,60];d5=[90,88,86];d6=[50,60,50];d7=[89,87];d8=[54,54];d9=[92,95,96,96,95,92,92];d10=[53,53,55,58,60,60,50];
      | 
      | 
      | elseif isequal(conntyp,'3 ports (primary grounded)')
      |     vin_sel=[1 2 5 3];
      |     Vinzeros=[0 0];
      |     hist_sel=[1 2 4];
      |   
      |      a1=0;a2=0;a3=100;a4=100; b1=[20,34,40,33,31,33,40,33,31,33,40,33,31,33,40,34,7];b2=[30,30,34,42,40,37,45,52,50,47,54,62,59,57,65,70,70];b3=[93,67,60,67,70,67,60,67,70,67,60,67,70,67,60,67,93];b4=[30,30,34,42,40,37,45,52,50,47,54,62,60,57,65,70,70];
      |     c1=[20,20];c2=[20,30];c3=[27,14];c4=[20,20];c5=[24,17];c6=[16,16];c7=[22,19];c8=[13,13];c9=[80,80]*0;c10=[20,30]*0;c11=[88,74]*0;c12=[20,20]*0;c13=[85,77]*0;c14=[16,16]*0;c15=[81,79]*0;c16=[13,13]*0;
      |     %d1=[85,80];d2=[60,60];d3=[83,83];d4=[50,60];d5=[90,88,86];d6=[50,60,50];d7=[89,87];d8=[54,54];d9=[92,95,96,96,95,92,92];d10=[53,53,55,58,60,60,50];
      | elseif isequal(conntyp,'3 ports (tapped secondary grounded)')
      |     vin_sel=[1 2 3 5];
      |     Vinzeros=[0 0];
      |     hist_sel=[1 2 3];
      |  
      |    a1=0;a2=0;a3=100;a4=100; b1=[20,34,40,33,31,33,40,33,31,33,40,33,31,33,40,34,7];b2=[30,30,34,42,40,37,45,52,50,47,54,62,59,57,65,70,70];b3=[80,67,60,67,70,67,60,67,70,67,60,67,70,67,60,67,93];b4=[30,30,34,42,40,37,45,52,50,47,54,62,60,57,65,70,70];
      |     c1=[20,20]*0;c2=[20,30]*0;c3=[27,14]*0;c4=[20,20]*0;c5=[24,17]*0;c6=[16,16]*0;c7=[22,19]*0;c8=[13,13]*0;c9=[80,80];c10=[20,30];c11=[88,74];c12=[20,20];c13=[85,77];c14=[16,16];c15=[81,79];c16=[13,13];
      |     %d1=[85,80];d2=[60,60];d3=[83,83];d4=[50,60];d5=[90,88,86];d6=[50,60,50];d7=[89,87];d8=[54,54];d9=[92,95,96,96,95,92,92];d10=[53,53,55,58,60,60,50];
      | elseif isequal(conntyp,'2 ports')
      |     vin_sel=[1 2 5 5];
      |     Vinzeros=[0 0 0];
      |     hist_sel=[1 2];
      |         a1=0;a2=0;a3=100;a4=100; b1=[20,34,40,33,31,33,40,33,31,33,40,33,31,33,40,34,7];b2=[30,30,34,42,40,37,45,52,50,47,54,62,59,57,65,70,70];b3=[80,67,60,67,70,67,60,67,70,67,60,67,70,67,60,67,93];b4=[30,30,34,42,40,37,45,52,50,47,54,62,60,57,65,70,70];
      |     c1=[20,20];c2=[20,30];c3=[27,14];c4=[20,20];c5=[24,17];c6=[16,16];c7=[22,19];c8=[13,13];c9=[80,80];c10=[20,30];c11=[88,74];c12=[20,20];c13=[85,77];c14=[16,16];c15=[81,79];c16=[13,13];
      |     %d1=[85,80];d2=[60,60];d3=[83,83];d4=[50,60];d5=[90,88,86];d6=[50,60,50];d7=[89,87];d8=[54,54];d9=[92,95,96,96,95,92,92];d10=[53,53,55,58,60,60,50];
      | else
      | 
      | end
      | 
      | ori=get_param(bloc,'Orientation');
      | 
      | if isequal(ori,'right')
      |     d1=[73,67];d2=[56,56];d3=[70,70];d4=[45,56];d5=[80,77,75];d6=[45,56,45];d7=[79,76];d8=[50,50];d9=[82,84,86,84,82,82];d10=[50,50,54,56,56,45];
      | else
      |     d1=[73,71,69,71,73,73];d2=[50,50,52,56,56,45];d3=[80,77,75];d4=[45,56,45];d5=[76,79];d6=[50,50];d7=[88,82];d8=[56,56];d9=[85,85];d10=[45,56];
      | end
      settings: LibrarySourceBlock=artemis/SSN/SSN OLTC/SSN OLTC xfo v2
      settings: CopyFcn=|
      | str=tempname;
      | str=strrep(str(end-20:end),'_','x');
      | set_param(gcb,'taggg',str);
      | set_param(gcb,'LinkStatus','inactive');
      mask Help: eval('open SSN_OLTC.pdf;');
      mask TypeOptions conntype: 4 ports | 3 ports (primary grounded) | 3 ports (tapped secondary grounded) | 2 ports
      mask Callback conntype:
      | bloc=gcb;
      | conntyp=get_param(bloc,'conntype');
      | nn=fts6_xfo_port_cb(bloc,conntyp);
      | set_param(bloc,'nnode',nn);
      mask Display:
      | plot(a1,a2,a3,a4,b1,b2,b3,b4,c1,c2,c3,c4,c5,c6,c7,c8,c9,c10,c11,c12,c13,c14,c15,c16);
      | color('blue');
      | plot(d1,d2,d3,d4,d5,d6,d7,d8,d9,d10);
  Transfo R2-L2-turnratio : Constant  Value=[0.0001 0.00001 1]
  x : Product  RndMeth=Zero
  L : PMIOPort  Tag=PMCPort  Side=Right
  S : PMIOPort  Port=2  Side=Left
  Isec : Outport
  Vsec : Outport  Port=2
  wires:
  Fcn/1 -> x/1
  Mux1/1 -> SSN OLTC xfo v2/1(params)
  x/1 -> Mux1/1
  Transfo R2-L2-turnratio/1 -> x/2
  Back-Euler/1 -> Mux1/2
  SSN OLTC xfo v2/1(meas) -> "   "/1  "transfo flux (Weber)"
  N/1 -> Fcn/1
  "    "/1 -> Memory1/1
  PT/1 -> "    "/1
  CT1/1 -> " 1"/1
  " 1"/1 -> Memory/1
  Memory1/1 -> Vsec/1
  Memory/1 -> Isec/1
  connections:
  CT1/RConn1 -- SSN Interface Block (1ph)2/RConn1 -- PT/LConn1
  SSN OLTC xfo v2/LConn1 -- SSN Interface Block (1ph)/RConn1
  SSN OLTC xfo v2/RConn1 -- SSN Interface Block (1ph)2/LConn1
  S/RConn1 -- SSN Interface Block (1ph)/LConn1
  PT/LConn2 -- Ground1/LConn1
  CT1/LConn1 -- L/RConn1

== system IEEE13bus_1subsystem/SM_13p/Regulator 1/Single Phase SVR_A/Voltage Regulator Control ==
  Vm : Inport
  Constant : Constant  Value=RegulatorOn
  Tap Changer Control : Subsystem  mask(Tap Changer Control){MinMaxTap=TapMinMax, InitialPosition=InitialTap, MecDelay=TapSelectionTime}
      mask prompts: MinMaxTap "Minimum and maximum tap number [ Min  Max ] :"; InitialPosition "Initial tap position"; MecDelay "Mechanical delay time"
      mask init:
      | if MecDelay<=0,
      | 	MecDelay=1/60;
      | end
  Voltage regulator : Subsystem  mask{Vref=RegulatorVref*120, DeadBand=RegulatorDeadBand*120, TimeDelay=RegulatorDelay}
      mask prompts: Vref "Vref (on 120v base)"; DeadBand "Deadband (on 120v base)"; TimeDelay "Time delay (s)"
  N : Outport
  Tap : Outport  Port=2
  wires:
  Voltage regulator/2(Down) -> Tap Changer Control/2("Down ")
  Tap Changer Control/1(TapNo) -> Tap/1, N/1  "Tap"
  Voltage regulator/1(Up) -> Tap Changer Control/1("Up ")
  Tap Changer Control/2(Ready) -> Voltage regulator/2(Ready)
  Constant/1 -> Voltage regulator/3(RegOn)
  Vm/1 -> Voltage regulator/1(Vmes (pu))

== system IEEE13bus_1subsystem/SM_13p/Regulator 1/Single Phase SVR_A1/Line Drop Compensator ==
  note: Vm=Vsec-Isec(Rc+jXc)
  Isec : Inport
  Vsec : Inport  Port=2
  "        " : spsLinearTransformerLib/Linear Transformer  UNITS=SI  NominalPower=[pNom fNom]  winding1=[vNom/ptRatio 1e-7 1e-8]  winding2=[vNom/ptRatio 1e-7 1e-8]  ThreeWindings=off  winding3=[3.15e+005 0.7938 0.084225]  RmLm=[1e5 1e5]  Measurements=None  DataType=on
  "CTS  " : spsControlledCurrentSourceLib/Controlled Current Source  Initialize=on  Source_Type=AC  Amplitude=0  Phase=0  Frequency=0  Measurements=None
  "PTS  " : spsControlledVoltageSourceLib/Controlled Voltage Source  Initialize=on  Source_Type=AC  Amplitude=0  Phase=0  Frequency=0  Measurements=None
  RMS : spsRMSLib/RMS  TrueRMS=on  Freq=60  RMSInit=120  Ts=0
  Raux : spsSeriesRLCBranchLib/Series RLC Branch  LConnTagsString=__new0  RConnTagsString=__new0  BranchType=R  Resistance=1e3  Inductance=1.6 / (120*pi)  SetiL0=off  InitialCurrent=0  Capacitance=1e-6  Setx0=off  InitialVoltage=0  Measurements=None
  Rc+jXc : spsSeriesRLCBranchLib/Series RLC Branch  LConnTagsString=__new0  RConnTagsString=__new0  BranchType=RL  Resistance=Rc  Inductance=Xc / (2*pi*fNom)  SetiL0=off  InitialCurrent=0  Capacitance=1e-6  Setx0=off  InitialVoltage=0  Measurements=None
  VRelay : spsVoltageMeasurementLib/Voltage Measurement  PhasorSimulation=off  OutputType=Complex  PSBequivalent=0
  Vm : Outport
  wires:
  RMS/1 -> Vm/1
  VRelay/1 -> RMS/1
  Isec/1 -> "CTS  "/1
  Vsec/1 -> "PTS  "/1
  connections:
  "PTS  "/RConn1 -- "        "/RConn1
  "        "/RConn2 -- VRelay/LConn1
  Raux/LConn1 -- Rc+jXc/LConn1 -- "        "/LConn1 -- "CTS  "/RConn1
  Rc+jXc/RConn1 -- Raux/RConn1 -- "CTS  "/LConn1 -- "        "/LConn2
  VRelay/LConn2 -- "PTS  "/LConn1
